simulink model "PID_Control_Wheel"  (R2017b)
settings: Solver=ode45  StartTime=0.0  StopTime=10.0  MaxStep=.01  RelTol=1e-3  EnableMultiTasking=on
values from neighbouring files (symbols this model uses):
  bw = 1    [Lab04_MATLAB_Script.m]
  CM = 1    [Lab04_MATLAB_Script.m]
  DCm = 2    [Lab04_MATLAB_Script.m]
  Disturbance = -5    [Lab04_MATLAB_Script.m]
  Jw = 4    [Lab04_MATLAB_Script.m]
  KD = 3    [Lab04_MATLAB_Script.m]
  KI = 2    [Lab04_MATLAB_Script.m]
  KP = 10    [Lab04_MATLAB_Script.m]
  r = 10    [Lab04_MATLAB_Script.m]
  taum = 0.5    [Lab04_MATLAB_Script.m]
  tdisturbance = 8    [Lab04_MATLAB_Script.m]
settings Model: Creator=rodrigue  LastModifiedBy=rodrigue
settings DataIOCC: SaveFormat=Array
settings OptimizationCC: LifeSpan=inf
settings DebuggingCC: SFUnexpectedBacktrackingDiag=warning  SFNoUnconditionalDefaultTransitionDiag=warning  SFExecutionAtInitializationDiag=none
settings HardwareCC: ProdBitPerPointer=32  ProdBitPerSizeT=32  ProdBitPerPtrDiffT=32  ProdLargestAtomicFloat=None  ProdIntDivRoundTo=Undefined  ProdEndianess=Unspecified  ProdWordSize=32  ProdHWDeviceType=32-bit Generic
settings ModelReferenceCC: PropagateSignalLabelsOutOfModel=off
settings CodeAppCC: StateflowObjectComments=on
settings GRTTargetCC: TargetLangStandard=C89/C90 (ANSI)  GeneratePreprocessorConditionals=Disable all
settings ConfigComp: CovMetricSettings=dw  CovHtmlReporting=on  CovSaveCumulativeToWorkspaceVar=on  CovSaveSingleToWorkspaceVar=on  CovExternalEMLEnable=off

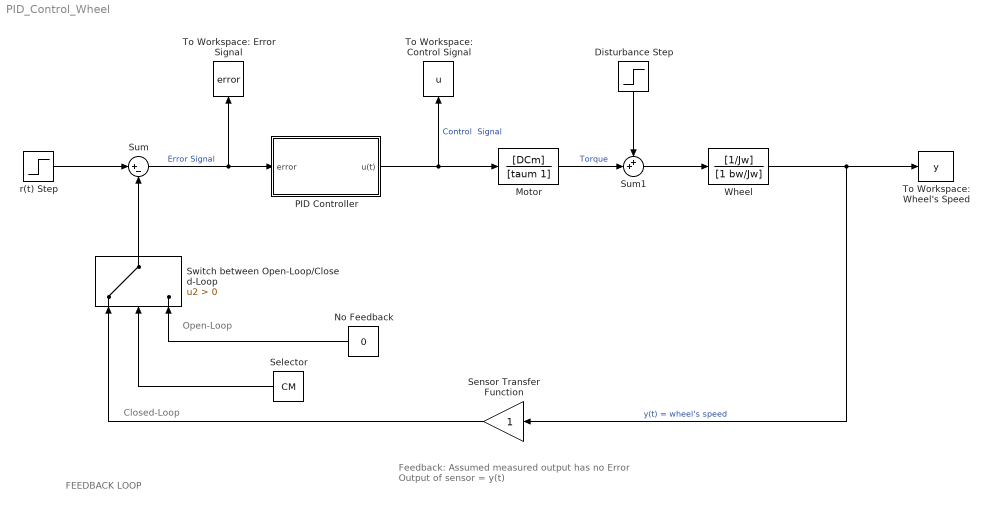
== system PID_Control_Wheel ==
  note: FEEDBACK LOOP
  note: Closed-Loop
  note: Open-Loop
  note: Feedback: Assumed measured output has no Error
      | Output of sensor = y(t)
  Disturbance Step : Step  Time=tdisturbance  After=Disturbance  SampleTime=0
  Motor : TransferFcn  Numerator=[DCm]  Denominator=[taum 1]
  No Feedback : Constant  Value=0
  PID Controller : Subsystem
  Selector : Constant  Value=CM
  Sensor Transfer Function : Gain
  Sum : Sum  Inputs=|+-
  Sum1 : Sum  Inputs=++|
  Switch between Open-Loop/Closed-Loop : Switch  Criteria=u2 > Threshold
  To Workspace: Control Signal : ToWorkspace  VariableName=u  SampleTime=-1
  To Workspace: Error Signal : ToWorkspace  VariableName=error  SampleTime=-1
  To Workspace: Wheel's Speed : ToWorkspace  VariableName=y  SampleTime=-1
  Wheel : TransferFcn  Numerator=[1/Jw]  Denominator=[1 bw/Jw]
  r(t) Step : Step  Time=0  After=r  SampleTime=0
  wires:
  Sum/1 -> PID Controller/1(error), To Workspace: Error Signal/1  "Error Signal"
  Wheel/1 -> Sensor Transfer Function/1, To Workspace: Wheel's Speed/1  "y(t) = wheel's speed"
  r(t) Step/1 -> Sum/1
  Switch between Open-Loop/Closed-Loop/1 -> Sum/2
  Motor/1 -> Sum1/2  "Torque"
  Sum1/1 -> Wheel/1
  Disturbance Step/1 -> Sum1/1
  PID Controller/1(u(t)) -> Motor/1, To Workspace: Control Signal/1  "Control  Signal"
  Selector/1 -> Switch between Open-Loop/Closed-Loop/2
  No Feedback/1 -> Switch between Open-Loop/Closed-Loop/3
  Sensor Transfer Function/1 -> Switch between Open-Loop/Closed-Loop/1

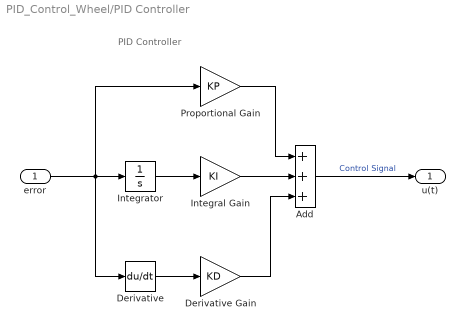
== system PID_Control_Wheel/PID Controller ==
  note: PID Controller
  error : Inport
  Add : Sum  Inputs=+++
  Derivative : Derivative
  Derivative Gain : Gain  Gain=KD
  Integral Gain : Gain  Gain=KI
  Integrator : Integrator
  Proportional Gain : Gain  Gain=KP
  u(t) : Outport
  wires:
  error/1 -> Derivative/1, Integrator/1, Proportional Gain/1
  Derivative/1 -> Derivative Gain/1
  Integrator/1 -> Integral Gain/1
  Integral Gain/1 -> Add/2
  Proportional Gain/1 -> Add/1
  Derivative Gain/1 -> Add/3
  Add/1 -> u(t)/1  "Control Signal"
